simulink model "MotDynoReferenceApplication"  (R2025a)
settings: Solver=VariableStepAuto  StartTime=0.0  StopTime=36  RelTol=1e-3
libraries: simulink x2, autolibinverter x2, autolibmotorctrlr x2, autolibpowerinfoutils x1, autolibpmsminterior x1, autolibfluxpmsm x1, autolibmappedmotor x1
(part 5 of 7)

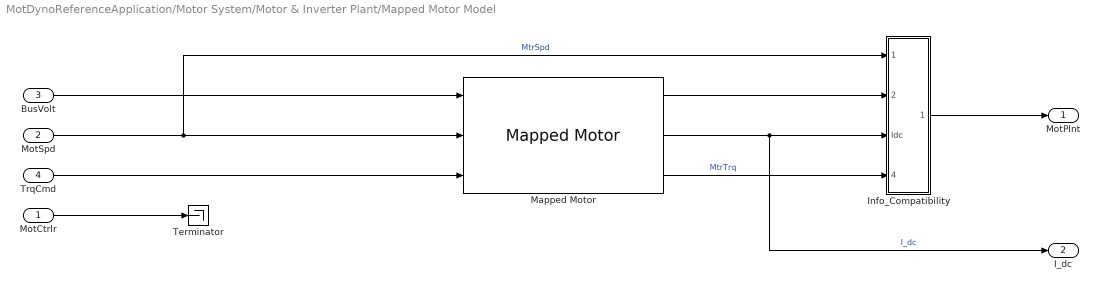
== system MotDynoReferenceApplication/Motor System/Motor & Inverter Plant/Mapped Motor Model ==
  MotCtrlr : Inport
  MotSpd : Inport  Port=2
  BusVolt : Inport  Port=3
  TrqCmd : Inport  Port=4
  Info_Compatibility : Subsystem
  Mapped Motor : autolibmappedmotor/Mapped Motor  w_Tmax_bp_ext=[-800;-750;-375;0;375;750;800]  Tmax_w_V_ext=[0 0 0;0.07 0.07 0.07;0.08 0.08 0.08;0.09 0.09 0.09;0.08 0.08 0.08;0.07 0.07 0.07;0 0 0]  w_Tmin_bp_ext=[-800;-750;-375;0;375;750;800]  Tmin_w_V_ext=[0 0 0;-0.07 -0.07 -0.07;-0.08 -0.08 -0.08;-0.09 -0.09 -0.09;-0.08 -0.08 -0.08;-0.07 -0.07 -0.07;0 0 0]  port_config=Speed  param_by=Tabulated torque-speed envelope  w_t=[0 167.55 335.1 468.94 502.65 670.21 837.76 1005.31 1172.86 1340.41 1507.96 1675.52]  T_t=[450 450 450 450 419.8 314.8 251.9 209.9 179.9 157.4 139.9 125.9]  torque_max=.1  power_max=30  SpreadsheetTqLimitsFileName=MotorCalibrationImportData.xlsx  Tmax_w_V=[0.09 0.09 0.09;0.08 0.08 0.08;0.07 0.07 0.07;0 0 0]  w_Tmax_bp=[ 0 375 750 800 ]  V_Tmax_bp=[500 750 900]  Tmin_w_V=[-0.09 -0.09 -0.09;-0.08 -0.08 -0.08;-0.07 -0.07 -0.07;0 0 0]  w_Tmin_bp=[ 0 375 750 800 ]  V_Tmin_bp=[500 750 900]  Tc=0.02  param_loss=Tabulated efficiency data  SpreadsheetLossFileName=MotorCalibrationImportData.xlsx  SpreadsheetEffFileName=MotorCalibrationImportData.xlsx  eff=100  w_eff=375  T_eff=0.08  Piron=0  Pbase=0  w_eff_bp=[0 167.55 335.1 468.94 502.65 670.21 837.76 1005.31 1172.86 1340.41 1507.96 1675.52]  T_eff_bp=[0 32.1 64.3 96.4 128.6 160.7 192.9 225 257.1 289.3 321.4 353.6 385.7 417.9 450]  Temp_eff_bp=[233.15 293.15 373.15]  V_eff_bp=[500 700 900]  losses_table=[1.49 1.67 2.21 3.10; 0.42 0.69 1.14 2.03; 0.06 0.24 0.78 1.68; 0.42 0.69 1.14 2.03; 1.49 1.67 2.21 3.10]  losses_table_3d=cat(3,[1.49 1.67 2.21 3.10; 0.42 0.69 1.14 2.03; 0.06 0.24 0.78 1.68; 0.42 0.69 1.14 2.03; 1.49 1.67 2.21 3.10],[1.49 1.67 2.21 3.10; 0.42 0.69 1.14 2.03; 0.06 0.24 0.78 1.68; 0.42 0.69 1.14 2.03; 1.49 1.67 2.21 3.10],[1.49 1.67 2.21 3.10; 0.42 0.69 1.14 2.03; 0.06 0.24 0.78 1.68; 0.42 0.69 1.14 2.03; 1.49 1.67 2.21 3.10])  losses_table_4d=cat(4,cat(3,[1.5645 0.441 0.063 0.441 1.5645;1.7535 0.7245 0.252 0.7245 1.7535;2.3205 1.197 0.819 1.197 2.3205;3.255 2.1315 1.764 2.1315 3.255],[1.5645 0.441 0.063 0.441 1.5645;1.7535 0.7245 0.252 0.7245 1.7535;2.3205 1.197 0.819 1.197 2.3205;3.255 2.1315 1.764 2.1315 3.255],[1.5645 0.441 0.063 0.441 1.5645;1.7535 0.7245 0.252 0.7245 1.7535;2.3205 1.197 0.819 1.197 2.3205;3.255 2.1315 1.764 2.1315 3.255]),cat(3,[1.49 0.42 0.06 0.42 1.49;1.67 0.69 0.24 0.69 1.67;2.21 1.14 0.78 1.14 2.21;3.1 2.03 1.68 2.03 3.1],[1.49 0.42 0.06 0.42 1.49;1.67 0.69 0.24 0.69 1.67;2.21 1.14 0.78 1.14 2.21;3.1 2.03 1.68 2.03 3.1],[1.49 0.42 0.06 0.42 1.49;1.67 0.69 0.24 0.69 1.67;2.21 1.14 0.78 1.14 2.21;3.1 2.03 1.68 2.03 3.1]),cat(3,[1.5347 0.4326 0.0618 0.4326 1.5347;1.7201 0.7107 0.2472 0.7107 1.7201;2.2763 1.1742 0.8034 1.1742 2.2763;3.193 2.0909 1.7304 2.0909 3.193],[1.5347 0.4326 0.0618 0.4326 1.5347;1.7201 0.7107 0.2472 0.7107 1.7201;2.2763 1.1742 0.8034 1.1742 2.2763;3.193 2.0909 1.7304 2.0909 3.193],[1.5347 0.4326 0.0618 0.4326 1.5347;1.7201 0.7107 0.2472 0.7107 1.7201;2.2763 1.1742 0.8034 1.1742 2.2763;3.193 2.0909 1.7304 2.0909 3.193]))  efficiency_table=[86.7 86.7 86.7 86.7 86.7 86.7 86.7 86.7 86.7 86.7 86.7 86.7 86.7 86.7 86.7;86.7 86.7 86.7 86.7 86.7 86.7 86.7 86.7 86.7 86.7 86.7 86.7 86.7 86.7 86.7;86.7 86.7 91.8 91.8 91.8 91.8 91.8 91.8 91.8 91.8 89.76 89.76 89.76 89.76 89.76;86.7 86.7 93.84 93.84 93.84 93.84 93.84 93.84 93.84 93.84 93.84 91.8 91.8 91.8 91.8;86.7 86.7 93.84 93.84 94.86 94.86 94.86 94.86 93.84 93.84 93.84 91.8 91.8 91.8 91.8;86.7 86.7 94.86 95.88 95.88 95.88 95.88 95.88 95.88 95.88 95.88 95.88 95.88 95.88 95.88;86.7 86.7 94.86 95.88 95.88 96.9 96.9 96.9 96.9 96.9 96.9 96.9 96.9 96.9 96.9;86.7 86.7 94.86 95.88 95.88 96.9 96.9 96.9 96.9 96.9 96.9 96.9 96.9 96.9 96.9;86.7 86.7 94.86 95.88 96.9 96.9 96.9 96.9 96.9 96.9 96.9 96.9 96.9 96.9 96.9;86.7 86.7 94.86 95.88 96.9 96.9 96.9 96.9 96.9 96.9 96.9 96.9 96.9 96.9 96.9;86.7 86.7 94.86 95.88 95.88 95.88 95.88 95.88 95.88 95.88 95.88 95.88 95.88 95.88 95.88;86.7 86.7 91.8 93.84 94.86 94.86 94.86 94.86 94.86 94.86 94.86 94.86 94.86 94.86 94.86]  efficiency_table_3d=cat(3,[95 95 95 95; 95 95 95 95; 95 95 95 95; 95 95 95 95; 95 95 95 95],[95 95 95 95; 95 95 95 95; 95 95 95 95; 95 95 95 95; 95 95 95 95],[95 95 95 95; 95 95 95 95; 95 95 95 95; 95 95 95 95; 95 95 95 95])  efficiency_table_4d=cat(4,cat(3,90*ones(5,4)',90*ones(5,4)',90*ones(5,4)'),cat(3,95*ones(5,4)',95*ones(5,4)',95*ones(5,4)'),cat(3,92*ones(5,4)',92*ones(5,4)',92*ones(5,4)'))  J=5e-6  b=1e-5  omega_o=0  T_t_extended=[125.9 139.9 157.4 179.9 209.9 251.9 314.8 419.8 450 450 450 450 450 450 450 419.8 314.8 251.9 209.9 179.9 157.4 139.9 125.9]  w_t_extended=[-1675.52 -1507.96 -1340.41 -1172.86 -1005.31 -837.76 -670.21 -502.65 -468.94 -335.1 -167.55 0 167.55 335.1 468.94 502.65 670.21 837.76 1005.31 1172.86 1340.41 1507.96 1675.52]  KLossIron=0  KLossCopper=0  x_w_eff_vec=[-1675.52 -1507.96 -1340.41 -1172.86 -1005.31 -837.76 -670.21 -502.65 -468.94 -335.1 -167.55 0 167.55 335.1 468.94 502.65 670.21 837.76 1005.31 1172.86 1340.41 1507.96 1675.52]  x_T_eff_vec=[-450 -417.9 -385.7 -353.6 -321.4 -289.3 -257.1 -225 -192.9 -160.7 -128.6 -96.4 -64.3 -32.1 0 32.1 64.3 96.4 128.6 160.7 192.9 225 257.1 289.3 321.4 353.6 385.7 417.9 450]  x_tmp_eff_vec=[-0.09 -0.06 -0.03 0 0.03 0.06 0.09]  x_V_eff_vec=[500 700 900]  x_losses_mat=[40854.7096774194 37940.4070537635 35017.0256057348 32102.7229820789 29179.3415340502 26265.0389103943 23341.6574623656 20427.3548387097 17513.0522150538 14589.6707670251 11675.3681433692 10602.7705507246 9623.4714074074 8250.63152941177 0 7153.297536 8834.34675199999 9949.6398848 11075.2542208 13839.7616896 16612.8813312 19377.3888 22141.8962688 24915.0159104 27679.5233792 30452.6430208 33217.1504896 35990.2701312 38754.7776;29158.9261576971 27078.9227584481 24992.4395978306 22912.4361985816 20825.9530379641 18745.9496387151 16659.4664780976 14579.4630788486 12499.4596795995 10412.9765189821 8332.973119733 6246.48995911556 5253.88779169303 7425.52898269897 0 6437.933628 4983.8379592 5989.1345728 7989.6546272 9983.9618864 11984.4819408 13978.7892 15973.0964592 17973.6165136 19967.9237728 21968.4438272 23962.7510864 25963.2711408 27957.5784;19296.9241486067 17920.4102260061 16539.6080980391 15163.0941754385 13782.2920474716 12405.7781248709 11024.975996904 9648.46207430336 8271.94815170275 6891.14602373578 5514.63210113516 5552.44012181894 4670.12635273035 6600.4756782007 0 5722.612413 4430.0818582 5323.6795888 5343.67850599999 6677.52049699998 8015.51775899998 9349.35974999997 10683.201741 12021.199003 13355.040994 14693.038256 16026.880247 17364.877509 18698.7194999999;16884.8266253869 15680.3756594427 14472.1725098039 13267.7215438596 12059.5183942208 10855.0674282765 9646.86427863773 8442.41331269346 7237.96234674919 6029.75919711039 4825.30823116613 4858.39028452232 4086.36491376766 5775.42237370242 0 5007.291198 3876.3257572 4658.2246048 4675.72367599999 5842.83666199998 7013.58551399998 8180.69849999998 9347.81148599998 10518.560338 11685.673324 12856.422176 14023.535162 15194.284014 16361.397;14472.7291021671 13440.3410928792 12404.7369215686 11372.3489122806 10336.74474097 9304.3567316821 8268.75256037148 7236.36455108356 6203.97654179564 5168.37237048501 5555.33383312474 4164.3404472257 3502.60347480498 4950.36906920415 0 4291.969983 3322.5696562 3992.7696208 5326.4540792 5008.15282699999 6011.65326899998 7012.03724999998 8012.42123099998 9015.92167299998 10016.305654 11019.806096 12020.190077 13023.690519 14024.0745;12060.6315789473 11200.3065263157 10337.3013333333 9476.97628070171 8613.97108771926 7753.64603508768 6890.64084210523 6030.31578947366 5169.99073684208 4306.98554385963 4629.45407092199 3470.29060992908 2918.8420358423 4125.31576470588 0 3576.648768 2768.8135552 3327.3146368 4438.7205632 4173.46899199999 5009.72102399999 5843.37599999998 6677.03097599998 7513.28300799998 8346.93798399998 9183.19001599998 10016.844992 10853.097024 11686.752;12959.6301627034 12035.1765444305 11107.8430083438 10183.3893900709 9256.05585398415 8331.60223571131 7404.26869962453 6479.81508135169 5555.36146307885 4628.02792699207 3703.57430871923 2776.24077263246 2335.08059687962 3300.26246020761 0 2861.327553 2215.0574542 2661.8596528 3550.9870472 4437.3531764 5326.4805708 6212.8467 7099.2128292 7988.3402236 8874.7063528 9763.8337472 10650.1998764 11539.3272708 12425.6934;20204.5588235294 18763.3002941176 17317.5518627451 15876.2933333333 10604.8437084399 9545.67916879796 8483.2150511509 6128.13330170779 5253.85295066415 4376.84898481974 3502.5686337761 3180.79319693095 2121.628657289 2475.15991349481 0 2145.963645 1990.936332 2984.856336 3322.536606 4151.878947 4983.804909 5813.14725 7960.649004 8957.665332 9951.585336 14574.43728 15897.51261 17224.70967 18547.785;18849.5490196078 17504.9478562091 16156.1579041394 14811.5567407407 9893.63455413471 8905.50241602729 7914.29198465474 6926.15984654732 5938.0277084399 4946.81727706735 3958.68513895993 2967.47470758739 1979.34256947997 2309.1644083045 0 2002.045542 1857.4150672 2784.6782656 3714.8301344 4642.0933328 5572.2452016 6499.5084 7426.7715984 8356.9234672 9284.1866656 13597.009088 14831.352956 16069.542132 17303.886;17202.9946524064 15975.8477005348 14744.8778609626 13517.7309090909 12286.7610695187 8659.52424836601 7695.69196078431 6734.85294117647 5774.01392156863 ...(+5339 chars)]  x_losses_mat_3d=[37.8947368421052 25.2631578947368 12.6315789473684 0 12 24 36;18.9473684210526 12.6315789473684 6.3157894736842 0 5.99999999999999 12 18;0 0 0 0 0 0 0;18 12 5.99999999999999 0 6.3157894736842 12.6315789473684 18.9473684210526;36 24 12 0 12.6315789473684 25.2631578947368 37.8947368421052]  x_losses_mat_4d="reshape([80;53.33;26.67;0;24;48;72;40;26.67;13.33;0;12;24;36;0;0;0;0;0;0;0;36;24;12;0;13.33;26.67;40;72;48;24;0;26.67;53.33;80;80;53.33;26.67;0;24;48;72;40;26.67;13.33;0;12;24;36;0;0;0;0;0;0;0;36;24;12;0;13.33;26.67;40;72;48;24;0;26.67;53.33;80;80;53.33;26.67;0;24;48;72;40;26.67;13.33;0;12;24;36;0;0;0;0;0;0;0;36;24;12;0;13.33;26.67;40;72;48;24;0;26.67;53.33;80;37.89;25.26;12.63;0;12;24;36;18.95;12.63;6.32;0;6;12;18;0;0;0;0;0;0;0;18;12;6;0;6.32;12.63;18.95;36;24;12;0;12.63;25.26;37.89;37.89;25.26;12.63;0;12;24;36;18.95;12.63;6.32;0;6;12;18;0;0;0;0;0;0;0;18;12;6;0;6.32;12.63;18.95;36;24;12;0;12.63;25.26;37.89;37.89;25.26;12.63;0;12;24;36;18.95;12.63;6.32;0;6;12;18;0;0;0;0;0;0;0;18;12;6;0;6.32;12.63;18.95;36;24;12;0;12.63;25.26;37.89;62.61;41.74;20.87;0;19.2;38.4;57.6;31.3;20.87;10.43;0;9.6;19.2;28.8;0;0;0;0;0;0;0;28.8;19.2;9.6;0;10.43;20.87;31.3;57.6;38.4;19.2;0;20.87;41.74;62.61;62.61;41.74;20.87;0;19.2;38.4;57.6;31.3;20.87;10.43;0;9.6;19.2;28.8;0;0;0;0;0;0;0;28.8;19.2;9.6;0;10.43;20.87;31.3;57.6;38.4;19.2;0;20.87;41.74;62.61;62.61;41.74;20.87;0;19.2;38.4;57.6;31.3;20.87;10.43;0;9.6;19.2;28.8;0;0;0;0;0;0;0;28.8;19.2;9.6;0;10.43;20.87;31.3;57.6;38.4;19.2;0;20.87;41.74;62.61], [7  5  3  3])"  CalLossMapData={}  CalLossWithTempMapData={}  aMode=6  RefBlkName='autolibmappedmotor/Mapped Motor'
  Terminator : Terminator
  MotPlnt : Outport  VectorParamsAs1DForOutWhenUnconnected=off
  I_dc : Outport  Port=2  VectorParamsAs1DForOutWhenUnconnected=off
  wires:
  MotCtrlr/1 -> Terminator/1
  MotSpd/1 -> Info_Compatibility/1(MtrSpd), Mapped Motor/2  "MtrSpd"
  BusVolt/1 -> Mapped Motor/1
  TrqCmd/1 -> Mapped Motor/3
  Mapped Motor/1 -> Info_Compatibility/2(Info)
  Mapped Motor/2 -> I_dc/1, Info_Compatibility/3(Idc)  "I_dc"
  Mapped Motor/3 -> Info_Compatibility/4(MtrTrq)  "MtrTrq"
  Info_Compatibility/1(Info_) -> MotPlnt/1
